simulink model "sim_test"  (R2022a)
settings: Solver=VariableStepAuto  StartTime=0.0  StopTime=10  RelTol=1e-3
values from neighbouring files (symbols this model uses):
  f0 = [0; 0; 0.5]    [SC_2DoF_Val_Init.m]    (also in sc_dyn_test.m; sc_spart_comp.m)
  n0 = [0; 0; 0]    [SC_2DoF_Val_Init.m]    (also in sc_dyn_test.m; sc_spart_comp.m)
  tau_qm = [0; 0]    [SC_2DoF_Val_Init.m]    (also in sc_dyn_test.m; sc_spart_comp.m)
libraries: robotmaniplib x5, SPART_Lib x1
settings Model: Creator=charl  LastModifiedBy=charl

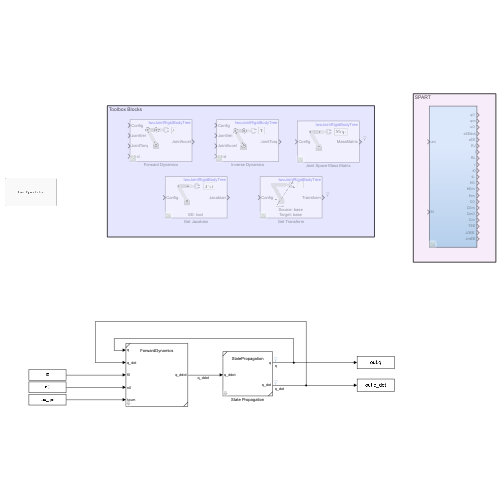
[thumbnail: Simulink's stored preview of the top-level diagram]
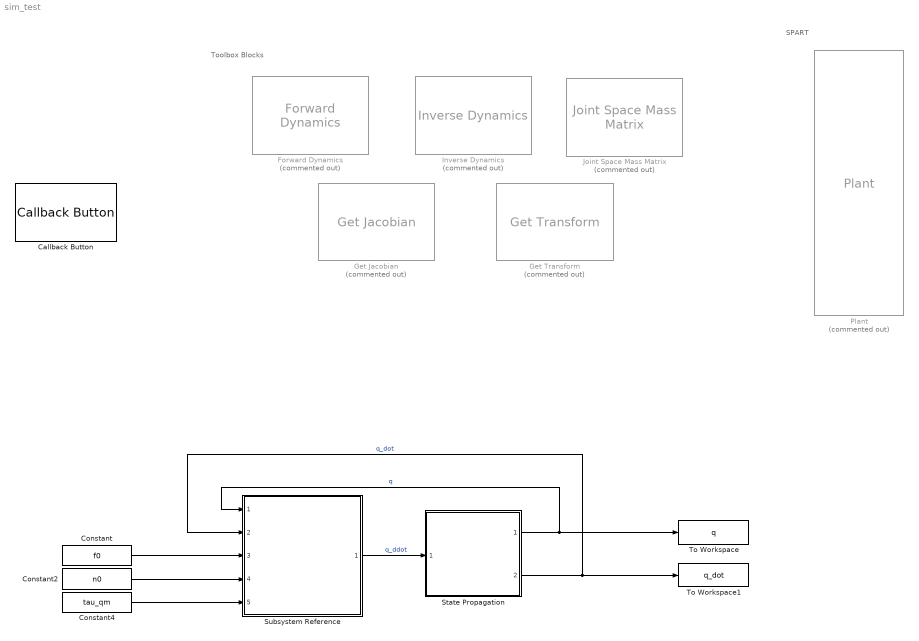
== system sim_test ==
  note: SPART
  note: Toolbox Blocks
  Callback Button : CallbackButton  ButtonText=Load SpaceRobot
      settings: ClickFcn=load('SC_2DoF.mat')
  Constant : Constant  Value=f0
  Constant2 : Constant  Value=n0
  Constant4 : Constant  Value=tau_qm
  Forward Dynamics : robotmaniplib/Forward Dynamics  Commented=on  RigidBodyTree=twoJointRigidBodyTree  SimulateUsing=Interpreted execution
  Get Jacobian : robotmaniplib/Get Jacobian  Commented=on  RigidBodyTree=twoJointRigidBodyTree  EndEffector=tool  SimulateUsing=Interpreted execution
      settings: SourceProductBaseCode=RO
  Get Transform : robotmaniplib/Get Transform  Commented=on  RigidBodyTree=twoJointRigidBodyTree  SourceBody=base  TargetBody=base  SimulateUsing=Interpreted execution
  Inverse Dynamics : robotmaniplib/Inverse Dynamics  Commented=on  RigidBodyTree=twoJointRigidBodyTree  SimulateUsing=Interpreted execution
      settings: SourceProductBaseCode=RO
  Joint Space Mass Matrix : robotmaniplib/Joint Space Mass Matrix  Commented=on  RigidBodyTree=twoJointRigidBodyTree  SimulateUsing=Interpreted execution
  Plant : SPART_Lib/Plant  Commented=on  SystemSampleTime=-1  VariantActivationTime=update diagram  Latency=0  AutoFrameSizeCalculation=off
  State Propagation : Subsystem  ReferencedSubsystem=StatePropagation  spaceRobot=sc
  Subsystem Reference : Subsystem  ReferencedSubsystem=ForwardDynamics  spaceRobot=sc  SimulateUsing=Interpreted execution
  To Workspace : ToWorkspace  VariableName=q  SaveFormat=Timeseries  SampleTime=-1
  To Workspace1 : ToWorkspace  VariableName=q_dot  SaveFormat=Timeseries  SampleTime=-1
  wires:
  Subsystem Reference/1 -> State Propagation/1  "q_ddot"
  Constant4/1 -> Subsystem Reference/5
  Constant2/1 -> Subsystem Reference/4
  Constant/1 -> Subsystem Reference/3
  State Propagation/1 -> Subsystem Reference/1, To Workspace/1  "q"
  State Propagation/2 -> Subsystem Reference/2, To Workspace1/1  "q_dot"
